simulink model "Wasing_machine"  (R2024a)
settings: Solver=VariableStepAuto  StartTime=0.0  StopTime=500  RelTol=1e-3
settings Model: Creator=Lenovo  LastModifiedBy=Lenovo

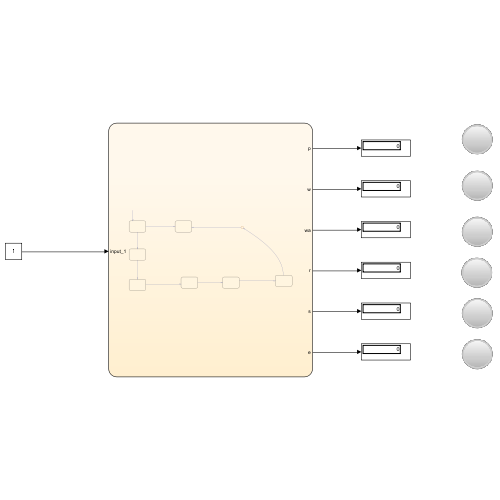
[thumbnail: Simulink's stored preview of the top-level diagram]
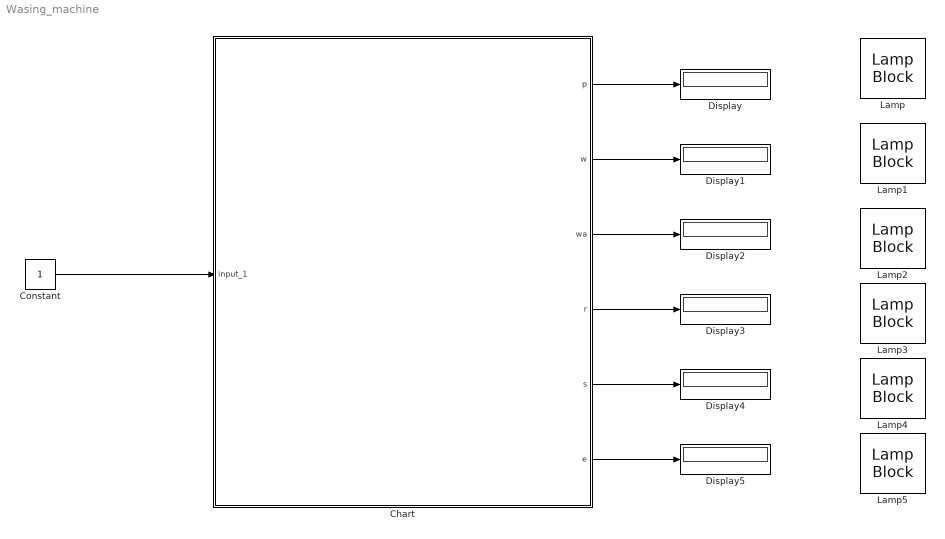
== system Wasing_machine ==
  Chart : Stateflow chart  TreatAsAtomicUnit=on
  Constant : Constant
  Display{,1..5} (6 alike) : Display
  Lamp{,1..5} (6 alike) : LampBlock  LabelPosition=Hide
  wires:
  Constant/1 -> Chart/1(input_1)
  Chart/6(e) -> Display5/1
  Chart/5(s) -> Display4/1
  Chart/4(r) -> Display3/1
  Chart/3(wa) -> Display2/1
  Chart/2(w) -> Display1/1
  Chart/1(p) -> Display/1

== stateflow chart Wasing_machine/Chart ==
  state power_on
    entry: p=1;
  state power_off
    entry:p=0;
  state water_fill
    entry:w=1;
  state done
    entry:e=1;
    exit:  e=0;
  state rinse
    entry: r=1;
    exit: r=0;
    entry: w=1;
  state spin
    entry: s=1;
    exit: s=0;
    entry: w=0;
  state wash
    entry: wa=1;
    exit: wa=0;
    entry: w=0;
  (default) -> power_on
  power_on -> power_off [order 2] : [input_1==0]
  (junction 10) -> power_off
  done -> (junction 10) : after(50,sec)
  power_on -> water_fill [order 1] : [input_1==1]
  water_fill -> wash : after(30,sec)
  spin -> done : after(50,sec)
  rinse -> spin : after(200,sec)
  wash -> rinse : after(100,sec)
  data: input_1 input; p output; w output; wa output; r output; s output; e output
